simulink model "w3prob1"  (R2020a)
settings: Solver=VariableStepAuto  StartTime=0.0  StopTime=10.0  RelTol=1e-3
settings Model: Creator=Anjali123  LastModifiedBy=Anjali123

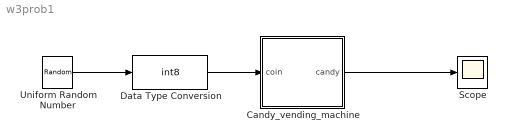
== system w3prob1 ==
  Candy_vending_machine : Stateflow chart  TreatAsAtomicUnit=on
  Data Type Conversion : DataTypeConversion  OutDataTypeStr=int8
  Scope : Scope
  Uniform Random Number : UniformRandomNumber  Minimum=0  Maximum=2  Seed=337  SampleTime=10
  wires:
  Uniform Random Number/1 -> Data Type Conversion/1
  Candy_vending_machine/1(candy) -> Scope/1
  Data Type Conversion/1 -> Candy_vending_machine/1(coin)

== stateflow chart w3prob1/Candy_vending_machine ==
  settings: stateMachineType=MEALY_MACHINE
  state Got_0
  state Got_1rupee
  state Got_2rupee
  (default) -> Got_0
  Got_0 -> Got_1rupee [order 1] : [coin == 1]{candy = 0;}
  Got_1rupee -> Got_0 [order 2] : [coin == 2]{candy = 1;}
  Got_0 -> Got_2rupee [order 2] : [coin == 2]{candy = 0;}
  Got_2rupee -> Got_0 [order 1] : [coin == 1]{candy = 1;}
  Got_2rupee -> Got_1rupee [order 2] : [coin == 2]{candy = 1;}
  Got_1rupee -> Got_2rupee [order 1] : [coin == 1]{candy = 0;}
  data: coin input; candy output
